simulink model "simVT2XC01_cruise"  (R2020b)
settings: Solver=VariableStepAuto  StartTime=0.0  StopTime=1000  RelTol=1e-3
undefined symbols (not defined in the file or in its folder): Ahrs, GPS, LineDispatcher, PhysicalState
libraries: aerolibactuator x4, mspsensorlib x1
settings Model: NumberOfSteps=5  Creator=test  LastModifiedBy=CHUNGNT28

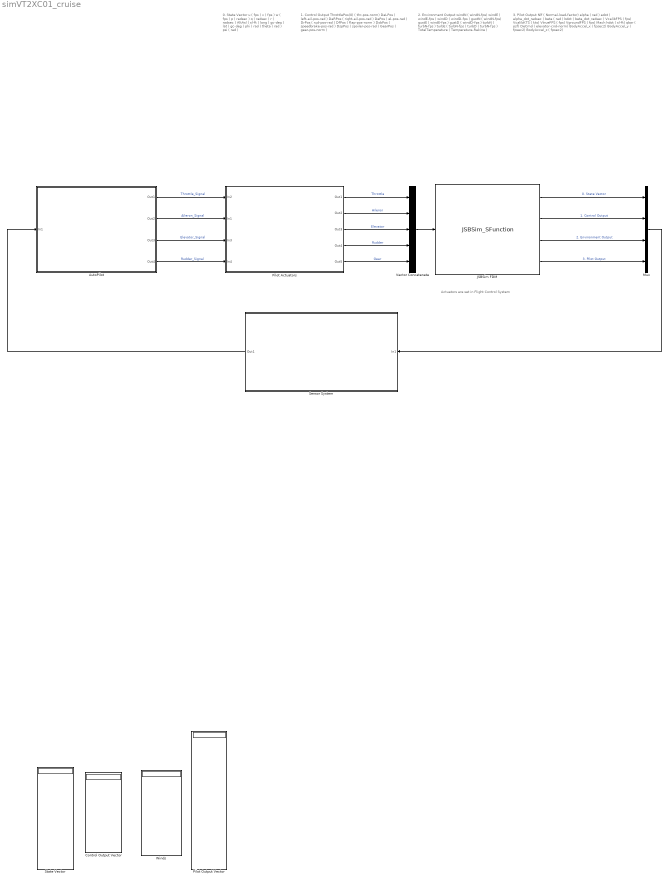
== system simVT2XC01_cruise ==
  note: 2. Environment Output
      |
      | windN ( windN-fps)
      | windE ( windE-fps )
      | windD ( windD-fps )
      | gustN ( windN-fps)
      | gustE ( windE-fps )
      | gustD ( windD-fps )
      | turbN ( turbN-fps )
      | turbE ( turbN-fps )
      | turbD ( turbN-fps )
      | TotalTemperature ( Temperature-Rakine )
  note: Actuators are set in Flight Control System
  note: 3. Pilot Output
      |
      | Nlf ( Normal-load-factor)
      | alpha ( rad )
      | adot ( alpha_dot_radsec )
      | beta ( rad )
      | bdot ( beta_dot_radsec )
      | VcalibFPS ( fps)
      | VcalibKTS ( kts)
      | VtrueFPS ( fps)
      | VgroundFPS ( fps)
      | Mach
      | hdot ( sl-ft)
      | qbar ( psf)
      | DeCmd ( elevator-cnd-norm)
      | BodyAccel_x ( fpsec2)
      | BodyAccel_y ( fpsec2)
      | BodyAccel_z ( fpsec2)
  note: 1. Control Output
      |
      | ThrottlePos(0) ( thr-pos-norm)
      | DaLPos ( left-ail-pos-rad )
      | DaRPos ( right-ail-pos-rad )
      | DePos ( el-pos-rad )
      | DrPos ( rud-pos-rad )
      | DfPos ( flap-pos-norm )
      | DsbPos ( speedbrake-pos-rad )
      | DspPos ( spoiler-pos-rad )
      | GearPos ( gear-pos-norm )
  note: 0. State Vector
      |
      | u ( fps )
      | v ( fps )
      | w ( fps )
      | p ( radsec )
      | q ( radsec )
      | r ( radsec )
      | AltAsl ( sl-ft )
      | long ( gc-deg )
      | lat ( gc-deg )
      | phi ( rad )
      | theta ( rad )
      | psi ( rad )
  AutoPilot : Subsystem  Tag=AutoPilot  Description=AutoPilot
      mask Display: image('C:\JSBSim\imgSys\autopilot.png'); % Use "Edit Image" on toolstrip to change.
  Control Output Vector : Display
  JSBSim FDM : S-Function  FunctionName=JSBSim_SFunction  Parameters='B747', In.init_params, In.init_pilotCmd, In.winds, [In.dt In.script_bool], 'scripts/B747_script1', '../../reset00'  SFunctionDeploymentMode=off  EnableBusSupport=off
      mask Display: image('C:\JSBSim\imgSys\logo_jsbsim_globe.svg'); % Use "Edit Image" on toolstrip to change.
  Mux : Mux
  Pilot Actuators : Subsystem
      mask Display: image('C:\JSBSim\imgSys\actuator_subsys.png'); % Use "Edit Image" on toolstrip to change.
  Pilot Output Vector : Display
  Sensor System : Subsystem
      mask Display: image('C:\JSBSim\imgSys\Sensor_subsys.png'); % Use "Edit Image" on toolstrip to change.
  State Vector : Display
  Vector Concatenate : Concatenate  NumInputs=5
  Winds : Display
  wires:
  Vector Concatenate/1 -> JSBSim FDM/1
  Pilot Actuators/2(Out2) -> Vector Concatenate/2  "Aileron"
  Pilot Actuators/4(Out4) -> Vector Concatenate/4  "Rudder"
  AutoPilot/1(Out1) -> Pilot Actuators/1(In2)  "Throttle_Signal"
  AutoPilot/2(Out2) -> Pilot Actuators/2(In1)  "Aileron_Signal"
  AutoPilot/3(Out3) -> Pilot Actuators/3(In3)  "Elevator_Signal"
  AutoPilot/4(Out4) -> Pilot Actuators/4(In4)  "Rudder_Signal"
  Pilot Actuators/1(Out1) -> Vector Concatenate/1  "Throttle"
  Pilot Actuators/3(Out3) -> Vector Concatenate/3  "Elevator"
  Pilot Actuators/5(Out5) -> Vector Concatenate/5  "Gear"
  JSBSim FDM/4 -> Mux/4  "3. Pilot Output"
  JSBSim FDM/3 -> Mux/3  "2. Environment Output"
  JSBSim FDM/2 -> Mux/2  "1. Control Output"
  JSBSim FDM/1 -> Mux/1  "0. State Vector"
  Mux/1 -> Sensor System/1(In1)
  Sensor System/1(Out1) -> AutoPilot/1(In1)

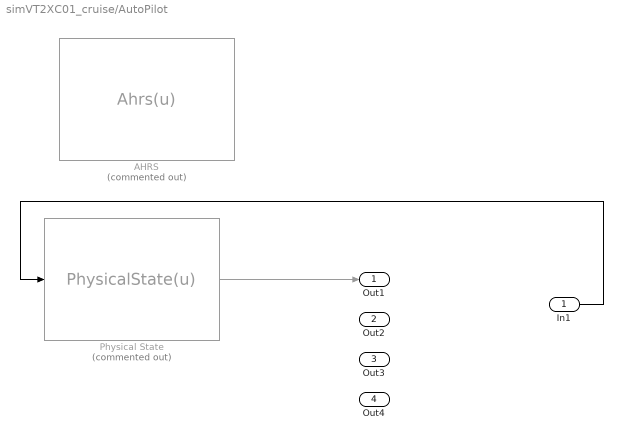
== system simVT2XC01_cruise/AutoPilot ==
  In1 : Inport
  AHRS : MATLABFcn  Commented=on  MATLABFcn=Ahrs(u)  OutputDimensions=1  SampleTime=0.01
      mask Display: image('C:\JSBSim\imgSys\ahrs.png'); % Use "Edit Image" on toolstrip to change.
  Physical State : MATLABFcn  Commented=on  MATLABFcn=PhysicalState(u)  OutputDimensions=1  SampleTime=0.01
      mask Display: image('C:\JSBSim\imgSys\PhysicalState.png'); % Use "Edit Image" on toolstrip to change.
  Out1 : Outport
  Out2 : Outport  Port=2
  Out3 : Outport  Port=3
  Out4 : Outport  Port=4
  wires:
  In1/1 -> Physical State/1
  Physical State/1 -> Out1/1

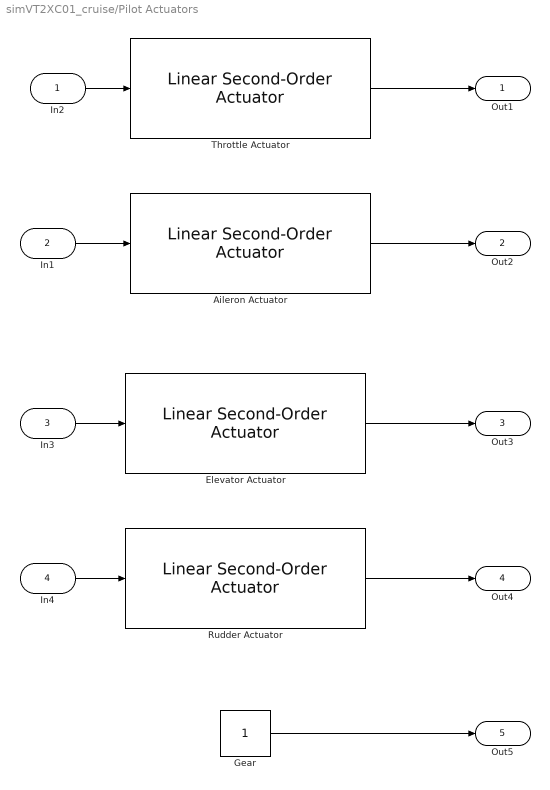
== system simVT2XC01_cruise/Pilot Actuators ==
  In2 : Inport
  In1 : Inport  Port=2
  In3 : Inport  Port=3
  In4 : Inport  Port=4
  Aileron Actuator : aerolibactuator/Linear Second-Order Actuator  wn_fin=1  z_fin=0.3  fin_act_0=0  fin_act_vel=0
      settings: SourceProductBaseCode=AE
  Elevator Actuator : aerolibactuator/Linear Second-Order Actuator  wn_fin=1  z_fin=0.3  fin_act_0=0  fin_act_vel=0
      settings: SourceProductBaseCode=AE
  Gear : Constant
  Rudder Actuator : aerolibactuator/Linear Second-Order Actuator  wn_fin=1  z_fin=0.3  fin_act_0=0  fin_act_vel=0
      settings: SourceProductBaseCode=AE
  Throttle Actuator : aerolibactuator/Linear Second-Order Actuator  wn_fin=1  z_fin=0.3  fin_act_0=0  fin_act_vel=0
      settings: SourceProductBaseCode=AE
  Out1 : Outport
  Out2 : Outport  Port=2
  Out3 : Outport  Port=3
  Out4 : Outport  Port=4
  Out5 : Outport  Port=5
  wires:
  In2/1 -> Throttle Actuator/1
  In1/1 -> Aileron Actuator/1
  In3/1 -> Elevator Actuator/1
  In4/1 -> Rudder Actuator/1
  Throttle Actuator/1 -> Out1/1
  Aileron Actuator/1 -> Out2/1
  Elevator Actuator/1 -> Out3/1
  Rudder Actuator/1 -> Out4/1
  Gear/1 -> Out5/1

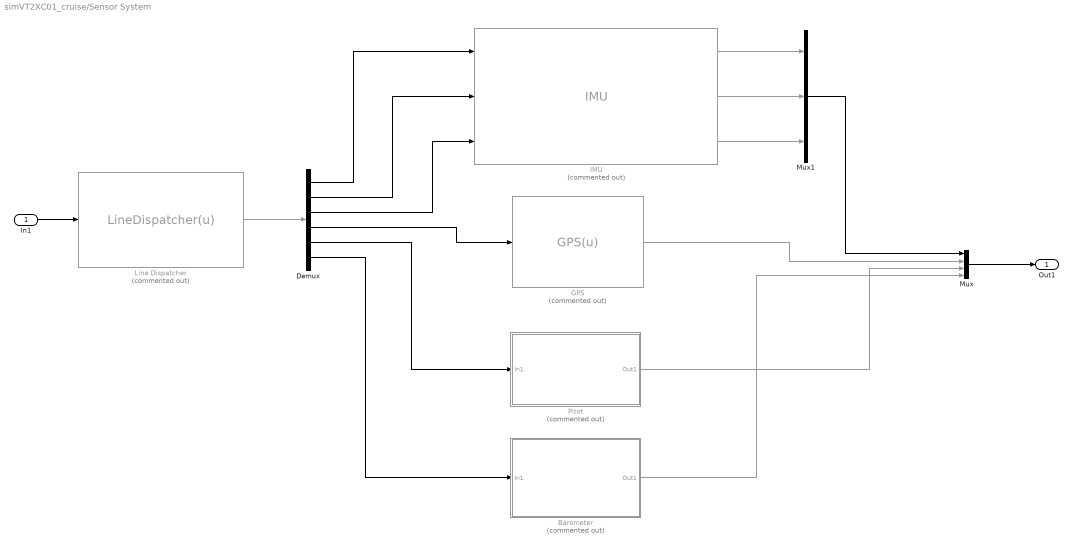
== system simVT2XC01_cruise/Sensor System ==
  In1 : Inport
  Barometer : Subsystem  Commented=on
      mask Display: image('C:\JSBSim\imgSys\BarometricPressureTempSensorICs.png'); % Use "Edit Image" on toolstrip to change.
  Demux : Demux  Outputs=[3 3 3 3 1 1]
  GPS : MATLABFcn  Commented=on  MATLABFcn=GPS(u)  OutputDimensions=1  SampleTime=0.01
      mask Display: image('C:\JSBSim\imgSys\gps_subsys.png'); % Use "Edit Image" on toolstrip to change.
  IMU : mspsensorlib/IMU  Commented=on  DispRefFrame=NED  Temperature=25  MagneticFieldNED=[ 27.5550, -2.4169, -16.0849 ]  MagneticFieldENU=[ -2.4169, 27.5550, 16.0849 ]  SeedDouble=67  SimulateUsing=Interpreted execution  AccelParamsMeasurementRange=accel.maxRead  AccelParamsResolution=accel.reso  AccelParamsConstantBias=accel.conOffBias  AccelParamsAxesMisalignment=accel.axesSkew  AccelParamsNoiseDensity=accel.noise.velRanWalk  AccelParamsBiasInstability=accel.noise.biasInstab  AccelParamsRandomWalk=accel.noise.accelRanWalk  AccelParamsTemperatureBias=accel.temEff.biasTem  AccelParamsTemperatureScaleFactor=accel.temEff.SF  GyroParamsMeasurementRange=gyro.maxRead  GyroParamsResolution=gyro.reso  GyroParamsConstantBias=gyro.conOffBias  GyroParamsAxesMisalignment=gyro.axesSkew  GyroParamsAccelerationBias=gyro.biasAccel  GyroParamsNoiseDensity=gyro.noise.angleRanWalk  GyroParamsBiasInstability=gyro.noise.biasInstab  GyroParamsRandomWalk=gyro.noise.rateRanWalk  GyroParamsTemperatureBias=gyro.temEff.biasTem  GyroParamsTemperatureScaleFactor=gyro.temEff.SF  MagParamsMeasurementRange=mag.maxRead  MagParamsResolution=mag.reso  MagParamsConstantBias=mag.conOffBias  MagParamsAxesMisalignment=mag.axesSkew  MagParamsNoiseDensity=mag.noise.whiteNoisePSD  MagParamsBiasInstability=mag.noise.biasInstab  MagParamsRandomWalk=mag.noise.ranWalk  MagParamsTemperatureBias=mag.temEff.biasTem  MagParamsTemperatureScaleFactor=mag.temEff.SF
      settings: SourceProductBaseCode=TF,NV
  Line Dispatcher : MATLABFcn  Commented=on  MATLABFcn=LineDispatcher(u)  OutputDimensions=4  SampleTime=0.01
      mask Display: image('$imagefile'); % Use "Edit Image" on toolstrip to change.
  Mux : Mux
  Mux1 : Mux  Inputs=3
  Pitot : Subsystem  Commented=on
      mask Display: image('C:\JSBSim\imgSys\pitot.png'); % Use "Edit Image" on toolstrip to change.
  Out1 : Outport
  wires:
  Mux/1 -> Out1/1
  IMU/2 -> Mux1/2
  IMU/3 -> Mux1/3
  IMU/1 -> Mux1/1
  Mux1/1 -> Mux/1
  GPS/1 -> Mux/2
  In1/1 -> Line Dispatcher/1
  Line Dispatcher/1 -> Demux/1
  Demux/1 -> IMU/1
  Demux/2 -> IMU/2
  Demux/3 -> IMU/3
  Demux/4 -> GPS/1
  Pitot/1(Out1) -> Mux/3
  Barometer/1(Out1) -> Mux/4
  Demux/5 -> Pitot/1(In1)
  Demux/6 -> Barometer/1(In1)

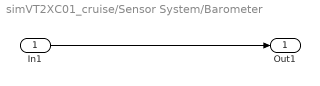
== system simVT2XC01_cruise/Sensor System/Barometer ==
  In1 : Inport
  Out1 : Outport
  wires:
  In1/1 -> Out1/1

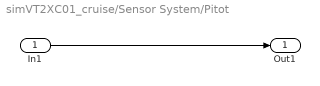
== system simVT2XC01_cruise/Sensor System/Pitot ==
  In1 : Inport
  Out1 : Outport
  wires:
  In1/1 -> Out1/1
